simulink model "PTODi_TrqDesCoord1"  (R2016b)
settings: configuration reference "CodeGenConfigSet" (kept outside this file)
values from neighbouring files (symbols this model uses):
  PT_trqCrSDCS_C = Calibration.Parameter    [init_PTODi_TrqDesCoord.m]    (also in init_PTODi_TrqDesCoord_SIL.m = Simulink.Parameter)
settings Model: Creator=Colin  LastModifiedBy=Wollf
settings ConfigSetRef: SourceLocation=Base Workspace

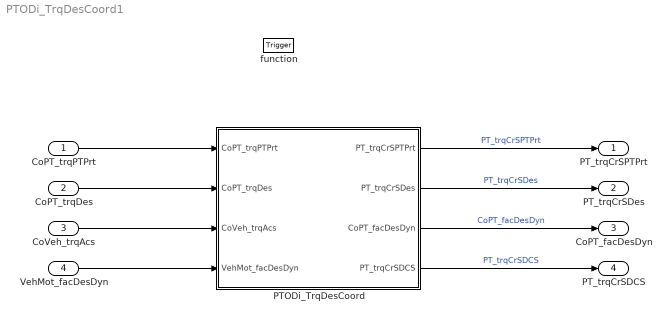
== system PTODi_TrqDesCoord1 ==
  CoPT_trqPTPrt : Inport  Tag=Nm  Description=Drive train protection torque (clutch torque)  OutMin=-3000  OutMax=3000  OutDataTypeStr=Trq_Nm
  CoPT_trqDes : Inport  Tag=Nm  Description=Total torque order for torque actuator (clutch torque)  Port=2  OutMin=-3000  OutMax=3000  OutDataTypeStr=Trq_Nm
  CoVeh_trqAcs : Inport  Tag=Nm  Description=message for demand of accessories  Port=3  OutMin=-3276.8  OutMax=3276.7  OutDataTypeStr=Trq_Nm
  VehMot_facDesDyn : Inport  Description=Dynamic factor for driver demand  Port=4  OutMin=-4  OutMax=3.999  OutDataTypeStr=Fact8192
  function : TriggerPort  TriggerType=function-call  VariantControl=Variant
  PTODi_TrqDesCoord : Subsystem
  PT_trqCrSPTPrt : Outport  Tag=Nm  Description=Application parameter for powertrain protection train protection torque(crankshaft torque)  OutMin=-3000  OutMax=3000  OutDataTypeStr=Trq_Nm
  PT_trqCrSDes : Outport  Tag=Nm  Description=Application parameter for requested propulsion torque to engine(crankshaft torque)  Port=2  OutMin=-3000  OutMax=3000  OutDataTypeStr=Trq_Nm
  CoPT_facDesDyn : Outport  Description=Dynamics factor of vehicle located requestors  Port=3  OutMin=-30  OutMax=30  OutDataTypeStr=Factor
  PT_trqCrSDCS : Outport  Tag=Nm  Description=crankshaft torque for request decrcment  Port=4  OutMin=-3000  OutMax=3000  OutDataTypeStr=Trq_Nm
  wires:
  PTODi_TrqDesCoord/1(PT_trqCrSPTPrt) -> PT_trqCrSPTPrt/1  "PT_trqCrSPTPrt"
  PTODi_TrqDesCoord/2(PT_trqCrSDes) -> PT_trqCrSDes/1  "PT_trqCrSDes"
  PTODi_TrqDesCoord/3(CoPT_facDesDyn) -> CoPT_facDesDyn/1  "CoPT_facDesDyn"
  VehMot_facDesDyn/1 -> PTODi_TrqDesCoord/4(VehMot_facDesDyn)
  CoVeh_trqAcs/1 -> PTODi_TrqDesCoord/3(CoVeh_trqAcs)
  CoPT_trqDes/1 -> PTODi_TrqDesCoord/2(CoPT_trqDes)
  CoPT_trqPTPrt/1 -> PTODi_TrqDesCoord/1(CoPT_trqPTPrt)
  PTODi_TrqDesCoord/4(PT_trqCrSDCS) -> PT_trqCrSDCS/1  "PT_trqCrSDCS"

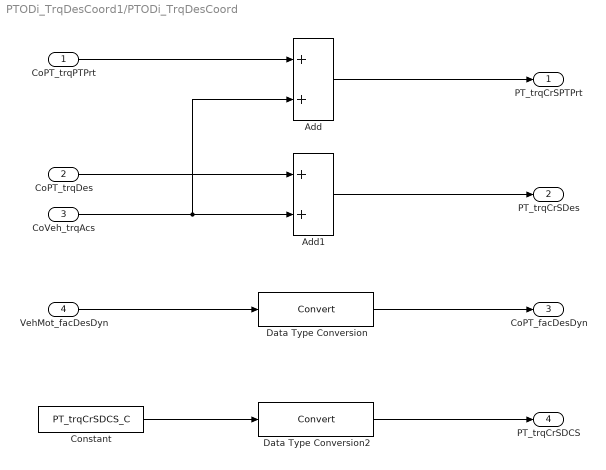
== system PTODi_TrqDesCoord1/PTODi_TrqDesCoord ==
  CoPT_trqPTPrt : Inport
  CoPT_trqDes : Inport  Port=2
  CoVeh_trqAcs : Inport  Port=3
  VehMot_facDesDyn : Inport  Port=4
  Add : Sum
  Add1 : Sum
  Constant : Constant  Value=PT_trqCrSDCS_C
  Data Type Conversion : DataTypeConversion
  Data Type Conversion2 : DataTypeConversion
  PT_trqCrSPTPrt : Outport
  PT_trqCrSDes : Outport  Port=2
  CoPT_facDesDyn : Outport  Port=3
  PT_trqCrSDCS : Outport  Port=4
  wires:
  CoPT_trqPTPrt/1 -> Add/1
  CoVeh_trqAcs/1 -> Add1/2, Add/2
  CoPT_trqDes/1 -> Add1/1
  Add1/1 -> PT_trqCrSDes/1
  Add/1 -> PT_trqCrSPTPrt/1
  Data Type Conversion/1 -> CoPT_facDesDyn/1
  VehMot_facDesDyn/1 -> Data Type Conversion/1
  Constant/1 -> Data Type Conversion2/1
  Data Type Conversion2/1 -> PT_trqCrSDCS/1
